simulink model "s2dot2_63jilianswitchfenduanhanshu"  (R2023b)
settings: Solver=VariableStepAuto  StartTime=0.0  StopTime=10  FixedStep=0.1  RelTol=1e-3
libraries: dspsrcs4 x1
settings Model: Creator=lxj  LastModifiedBy=lxj
settings DataIOCC: ExternalInput=t

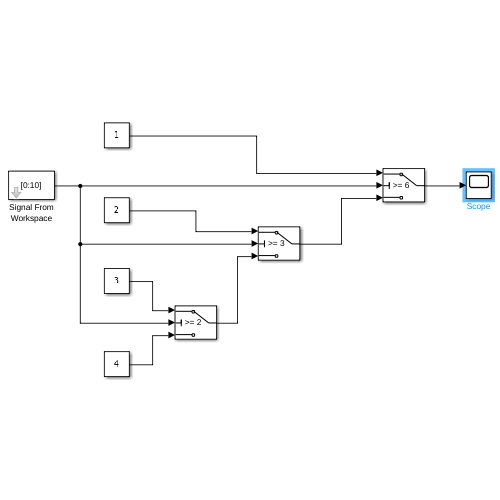
[thumbnail: Simulink's stored preview of the top-level diagram]
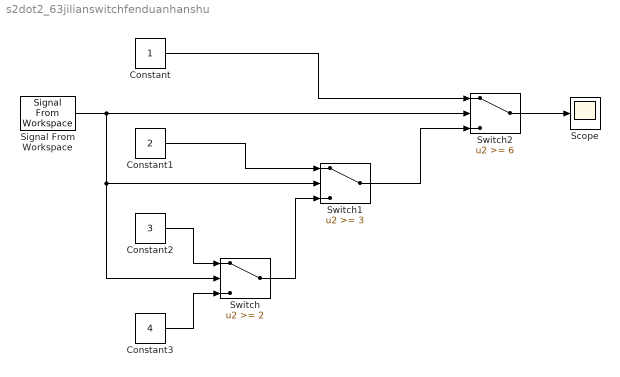
== system s2dot2_63jilianswitchfenduanhanshu ==
  Constant : Constant
  Constant1 : Constant  Value=2
  Constant2 : Constant  Value=3
  Constant3 : Constant  Value=4
  Scope : Scope
  Signal From Workspace : dspsrcs4/Signal From Workspace  X=[0:10]  Ts=1  nsamps=1  OutputAfterFinalValue=Setting to zero  ignoreOrWarnInputAndFrameLengths=on  OutputFrames=off
  Switch : Switch  Threshold=2  ZeroCross=off  SaturateOnIntegerOverflow=off  InputSameDT=off
  Switch1 : Switch  Threshold=3  ZeroCross=off  SaturateOnIntegerOverflow=off  InputSameDT=off
  Switch2 : Switch  Threshold=6  ZeroCross=off  SaturateOnIntegerOverflow=off  InputSameDT=off
  wires:
  Switch2/1 -> Scope/1
  Constant/1 -> Switch2/1
  Constant1/1 -> Switch1/1
  Constant3/1 -> Switch/3
  Constant2/1 -> Switch/1
  Switch/1 -> Switch1/3
  Switch1/1 -> Switch2/3
  Signal From Workspace/1 -> Switch/2, Switch1/2, Switch2/2
